simulink model "sensorTemperature"  (R2023a)
settings: Solver=VariableStepAuto  StartTime=0.0  StopTime=10.0  RelTol=1e-3
settings Model: Creator=rafael  LastModifiedBy=rafael

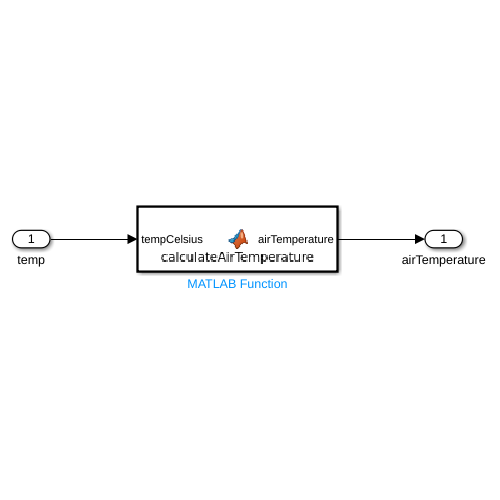
[thumbnail: Simulink's stored preview of the top-level diagram]
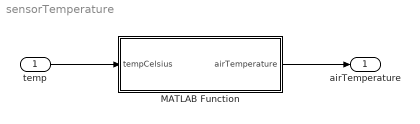
== system sensorTemperature ==
  temp : Inport
  MATLAB Function : MATLAB Function  TreatAsAtomicUnit=on
  airTemperature : Outport
  wires:
  temp/1 -> MATLAB Function/1(tempCelsius)
  MATLAB Function/1(airTemperature) -> airTemperature/1

== matlab function sensorTemperature/MATLAB Function ==
  data: tempCelsius input; airTemperature output
function airTemperature = calculateAirTemperature(tempCelsius)
    % FUNCTION Calculate Air Tempperature [K]
    airTemperature = tempCelsius*10; 
end
